simulink model "prelab"  (R2022a)
settings: Solver=VariableStepAuto  StartTime=0.0  StopTime=10  RelTol=1e-3
undefined symbols (not defined in the file or in its folder): A1, A2, A3, B1, B2, B3, F1, F2, F3
settings Model: Creator=varunsampat  LastModifiedBy=vishn
settings DebuggingCC: UnconnectedInputMsg=warning  UnconnectedOutputMsg=warning  UnconnectedLineMsg=warning
settings RTWCC: DLArmComputeVersion=19.05

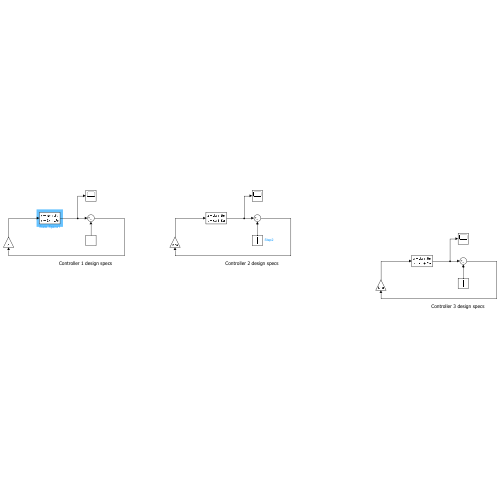
[thumbnail: Simulink's stored preview of the top-level diagram]
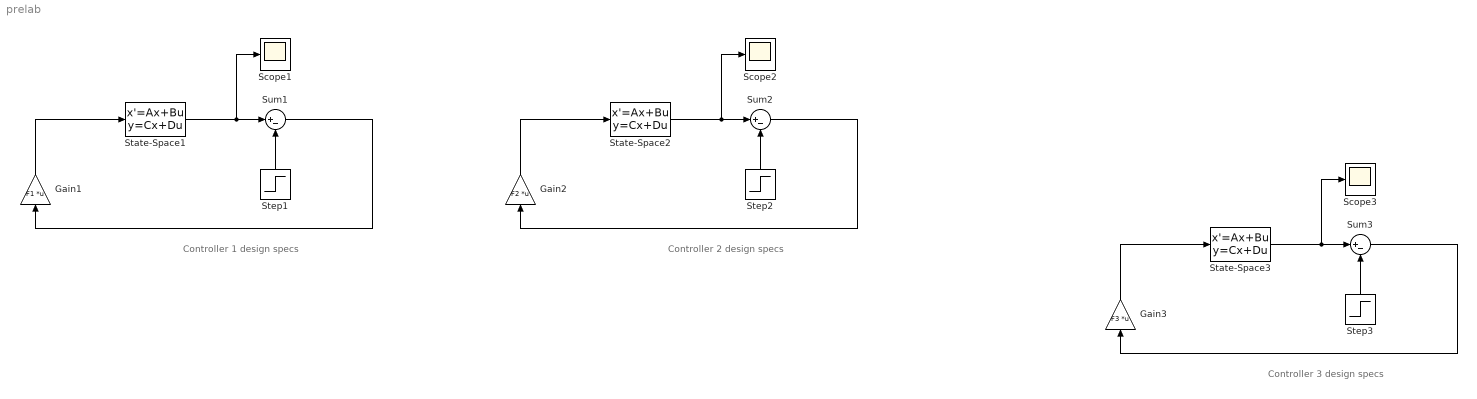
== system prelab ==
  note: Controller 1 design specs
  note: Controller 2 design specs
  note: Controller 3 design specs
  Gain1 : Gain  Gain=F1  Multiplication=Matrix(K*u)
  Gain2 : Gain  Gain=F2  Multiplication=Matrix(K*u)
  Gain3 : Gain  Gain=F3  Multiplication=Matrix(K*u)
  Scope1 : Scope
  Scope2 : Scope
  Scope3 : Scope
  State-Space1 : StateSpace  A=A1  B=B1  C=eye(4)  D=zeros(4,1)  InitialCondition=[0;0;0;0]
  State-Space2 : StateSpace  A=A2  B=B2  C=eye(4)  D=zeros(4,1)  InitialCondition=[0;0;0;0]
  State-Space3 : StateSpace  A=A3  B=B3  C=eye(4)  D=zeros(4,1)  InitialCondition=[0;0;0;0]
  Step1 : Step  Before=[0; 0; 0; 0]  After=[1; 0; 0; 0]  SampleTime=0
  Step2 : Step  Before=[0; 0; 0; 0]  After=[1; 0; 0; 0]  SampleTime=0
  Step3 : Step  Before=[0; 0; 0; 0]  After=[1; 0; 0; 0]  SampleTime=0
  Sum1 : Sum  Inputs=|+-
  Sum2 : Sum  Inputs=|+-
  Sum3 : Sum  Inputs=|+-
  wires:
  Gain1/1 -> State-Space1/1
  State-Space1/1 -> Scope1/1, Sum1/1
  Step1/1 -> Sum1/2
  Sum1/1 -> Gain1/1
  Sum2/1 -> Gain2/1
  Gain2/1 -> State-Space2/1
  Step2/1 -> Sum2/2
  State-Space2/1 -> Scope2/1, Sum2/1
  State-Space3/1 -> Scope3/1, Sum3/1
  Sum3/1 -> Gain3/1
  Step3/1 -> Sum3/2
  Gain3/1 -> State-Space3/1
